simulink model "FP_250521"  (R2024a)
settings: Solver=VariableStepAuto  StartTime=0.0  StopTime=10.0  RelTol=1e-3
values from neighbouring files (symbols this model uses):
  global_path_xy_dense = [-80.8928520527 -80.3602143869 -79.8516651737 -79.3645247642 -78.8961135098 -78.4437517617 -78.004759871 -77.5764581893 -77.1561670675 -76.7412068571 -76.3288979094 -75.9165605754 ... (728 elements, 364x2)]    [global_path_xy_dense_y-34.mat]
undefined symbols (not defined in the file or in its folder): Do_waypoints, do_waypoints_tail_shifted, pathXY, route1_waypoint, route1_waypoint_raw, route2_waypoint, route2_waypoint_raw, route3_waypoint, route3_waypoint_raw
libraries: CarMaker4SL x192, slpidlib x4
(part 2 of 4)

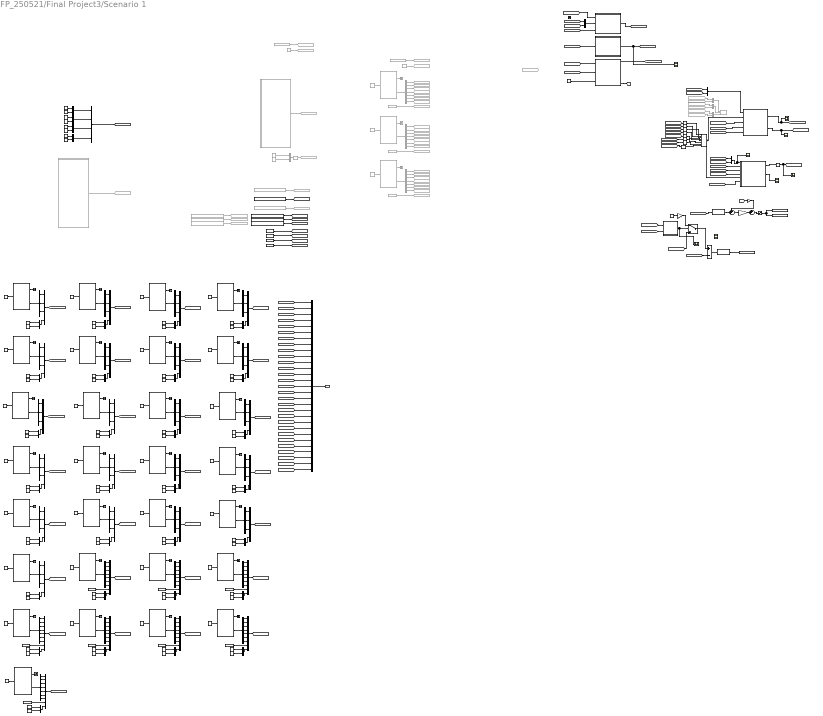
== system FP_250521/Final Project3/Scenario 1 ==
  note: 주차장 들어가기 전, 참이면 1 ==정지
  note: 적분기 출력 제한 -1~1
  note: 주차 경로 개인
  note: 주행 개인
  note: Traffic Size
      | Length: 4.47
      | Width: 1.97
      | Height: 1.12
  note: Traffic Size
      | Length: 4.47
      | Width: 1.97
      | Height: 1.12
  note: Traffic Size
      | Length: 4.47
      | Width: 1.97
      | Height: 1.12
  note: Traffic Size
      | Length: 4.47
      | Width: 1.97
      | Height: 1.12
  note: Traffic Size
      | Length: 4.47
      | Width: 1.97
      | Height: 1.12
  note: Traffic Size
      | Length: 4.47
      | Width: 1.97
      | Height: 1.12
  note: Traffic Size
      | Length: 4.47
      | Width: 1.97
      | Height: 1.12
  note: Traffic Size
      | Length: 4.47
      | Width: 1.97
      | Height: 1.12
  note: Traffic Size
      | Length: 4.47
      | Width: 1.97
      | Height: 1.12
  note: Traffic Size
      | Length: 4.47
      | Width: 1.97
      | Height: 1.12
  note: Traffic Size
      | Length: 4.47
      | Width: 1.97
      | Height: 1.12
  note: Traffic Size
      | Length: 4.47
      | Width: 1.97
      | Height: 1.12
  note: Traffic Size
      | Length: 4.47
      | Width: 1.97
      | Height: 1.12
  note: Traffic Size
      | Length: 4.47
      | Width: 1.97
      | Height: 1.12
  note: Traffic Size
      | Length: 4.47
      | Width: 1.97
      | Height: 1.12
  note: Traffic Size
      | Length: 4.47
      | Width: 1.97
      | Height: 1.12
  note: Traffic Size
      | Length: 4.47
      | Width: 1.97
      | Height: 1.12
  note: Traffic Size
      | Length: 4.47
      | Width: 1.97
      | Height: 1.12
  note: Traffic Size
      | Length: 4.47
      | Width: 1.97
      | Height: 1.12
  note: Traffic Size
      | Length: 4.47
      | Width: 1.97
      | Height: 1.12
  note: Traffic Size
      | Length: 4.47
      | Width: 1.97
      | Height: 1.12
  note: Traffic Size
      | Length: 4.47
      | Width: 1.97
      | Height: 1.12
  note: Traffic Size
      | Length: 4.47
      | Width: 1.97
      | Height: 1.12
  note: Traffic Size
      | Length: 4.47
      | Width: 1.97
      | Height: 1.12
  note: Traffic Size
      | Length: 4.47
      | Width: 1.97
      | Height: 1.12
  note: Traffic Size
      | Length: 4.47
      | Width: 1.97
      | Height: 1.12
  note: Traffic Size
      | Length: 4.47
      | Width: 1.97
      | Height: 1.12
  note: Traffic Size
      | Length: 4.47
      | Width: 1.97
      | Height: 1.12
  note: Traffic Size
      | Length: 4.47
      | Width: 1.97
      | Height: 1.12
  note: Do Not Modify !!
  note: *** Final Project ***
      |
      | Scenario:
      | Input:
      | Output:
      | 제어기 10ms / 다익스트라 1s
  note: Traffic Size
      | Length: 4.47
      | Width: 1.97
      | Height: 1.12
  note: Traffic Size
      | Length: 4.47
      | Width: 1.97
      | Height: 1.12
  note: Modify !!
  note: Traffic Size
      | Length: 4.47
      | Width: 1.97
      | Height: 1.12
  note: Do Not Modify !!
  note: Average Filter
  Add : Sum  Inputs=+-
  Bus Selector : BusSelector  Commented=on  OutputSignals=t_0 x,t_0 y,v_0 x,v_0 y,a_0 x,a_0 y,r_zyx z
  Bus Selector1 : BusSelector  Commented=on  OutputSignals=t_0 x,t_0 y,v_0 x,v_0 y,a_0 x,a_0 y,r_zyx z
  Bus Selector{3..19,22,28..30} (21 alike) : BusSelector  OutputSignals=t_0 x,t_0 y,r_zyx z
  Bus Selector2 : BusSelector  Commented=on  OutputSignals=t_0 x,t_0 y,v_0 x,v_0 y,a_0 x,a_0 y,r_zyx z
  Bus Selector{20..21,23..27,31} (8 alike) : BusSelector  OutputSignals=t_0 x,t_0 y,v_0 x,v_0 y,a_0 x,a_0 y,r_zyx z
  Constant : Constant  Commented=on  Value=80
  Constant1 : Constant  Commented=on  Value=0
  Constant10 : Constant  Commented=on  Value=2.48
  Constant100 : Constant  Value=47.5
  Constant101 : Constant  Value=-45
  Constant102 : Constant  Value=5.5
  Constant103 : Constant  Value=-45
  Constant104 : Constant  Value=47.5
  Constant105 : Constant  Value=-4
  Constant106 : Constant  Commented=on  Value=pathXY
  Constant107 : Constant  Commented=on  Value=route1_waypoint
  Constant108 : Constant  Commented=on  Value=route2_waypoint
  Constant109 : Constant  Commented=on  Value=route3_waypoint
  Constant11 : Constant
  Constant110 : Constant  Value=global_path_xy_dense
  Constant111 : Constant  Commented=on  Value=Do_waypoints
  Constant112 : Constant
  Constant12 : Constant  Value=5
  Constant{13,16,19,21..22,26,29,32,35,39,42,46,48,52,55..56,59,61,65,69,72,74,79,82,85,87..88,92,96} (29 alike) : Constant  Value=4.47
  Constant{14,17,23..24,27,30,33,36..37,40,43,49..50,53,57,62..63,66..67,70,75..76,80,83,89..90,93..94,97} (29 alike) : Constant  Value=1.97
  Constant15 : Constant  Value=7
  Constant18 : Constant  Value=8
  Constant2 : Constant  Commented=on
  Constant20 : Constant  Value=4
  Constant25 : Constant  Value=10
  Constant28 : Constant  Value=11
  Constant3 : Constant  Commented=on  Value=2
  Constant31 : Constant  Value=12
  Constant34 : Constant  Value=9
  Constant38 : Constant  Value=14
  Constant4 : Constant  Commented=on  Value=80
  Constant41 : Constant  Value=15
  Constant44 : Constant  Value=2
  Constant45 : Constant  Value=16
  Constant47 : Constant  Value=13
  Constant5 : Constant  Commented=on  Value=11.5
  Constant51 : Constant  Value=18
  Constant54 : Constant  Value=19
  Constant58 : Constant  Value=6
  Constant6 : Constant  Value=route1_waypoint_raw
  Constant60 : Constant  Value=17
  Constant64 : Constant  Value=21
  Constant68 : Constant  Value=22
  Constant7 : Constant
  Constant71 : Constant  Value=23
  Constant73 : Constant  Value=20
  Constant77 : Constant  Value=3
  Constant78 : Constant  Value=25
  Constant8 : Constant  Value=route2_waypoint_raw
  Constant81 : Constant  Value=26
  Constant84 : Constant  Value=27
  Constant86 : Constant  Value=24
  Constant9 : Constant  Value=route3_waypoint_raw
  Constant91 : Constant  Value=0
  Constant95 : Constant  Value=28
  Constant98 : Constant  Value=5.5
  Constant99 : Constant  Value=-4
  From2 : From  Commented=on  GotoTag=Global_Waypoints2
  From28 : From  Commented=on  GotoTag=Traffic00_Global_X
  From29 : From  Commented=on  GotoTag=Traffic00_Global_Y
  From30 : From  Commented=on  GotoTag=Traffic01_Global_X
  From31 : From  Commented=on  GotoTag=Traffic01_Global_Y
  From32 : From  Commented=on  GotoTag=Traffic02_Global_X
  From33 : From  Commented=on  GotoTag=Traffic02_Global_Y
  Gain : Gain  Gain=pi/180
  Gain1 : Gain  Gain=3
  Gain2 : Gain  Gain=0
  Goto1 : Goto  Commented=on  GotoTag=CrossTrackError
  Goto10 : Goto  Commented=on  GotoTag=Traffic00_Yaw
  Goto11 : Goto  Commented=on  GotoTag=Traffic01_Yaw
  Goto12 : Goto  Commented=on  GotoTag=Traffic01_YawRate
  Goto13 : Goto  Commented=on  GotoTag=Traffic01_Global_X
  Goto14 : Goto  Commented=on  GotoTag=Traffic01_Global_Y
  Goto15 : Goto  Commented=on  GotoTag=Traffic01_Vx
  Goto16 : Goto  Commented=on  GotoTag=Traffic01_Vy
  Goto17 : Goto  Commented=on  GotoTag=Traffic01_Ax
  Goto18 : Goto  Commented=on  GotoTag=Traffic01_Ay
  Goto19 : Goto  Commented=on  GotoTag=Traffic02_Yaw
  Goto2 : Goto  Commented=on  GotoTag=Traffic00_YawRate
  Goto20 : Goto  Commented=on  GotoTag=Traffic02_YawRate
  Goto21 : Goto  Commented=on  GotoTag=Traffic02_Global_X
  Goto22 : Goto  Commented=on  GotoTag=Traffic02_Global_Y
  Goto23 : Goto  Commented=on  GotoTag=Traffic02_Vx
  Goto24 : Goto  Commented=on  GotoTag=Traffic02_Vy
  Goto25 : Goto  Commented=on  GotoTag=Traffic02_Ax
  Goto26 : Goto  Commented=on  GotoTag=Traffic02_Ay
  Goto27 : Goto  Commented=on  GotoTag=CrossTrackError
  Goto28 : Goto  Commented=on  GotoTag=Traffic_size
  Goto29 : Goto  Commented=on  GotoTag=Target_Speed
  Goto3 : Goto  Commented=on  GotoTag=Traffic00_Global_X
  Goto30 : Goto  Commented=on  GotoTag=Traffic_Info
  Goto4 : Goto  Commented=on  GotoTag=Target_Speed
  Goto5 : Goto  Commented=on  GotoTag=Traffic00_Global_Y
  Goto6 : Goto  Commented=on  GotoTag=Traffic00_Vx
  Goto7 : Goto  Commented=on  GotoTag=Traffic00_Vy
  Goto73 : Goto  Commented=on  GotoTag=Global_Waypoints4
  Goto75 : Goto  Commented=on  GotoTag=Obstacle_Info
  Goto76 : Goto  Commented=on  GotoTag=Global_Waypoints1
  Goto77 : Goto  Commented=on  GotoTag=Global_Waypoints2
  Goto78 : Goto  Commented=on  GotoTag=Global_Waypoints3
  Goto8 : Goto  Commented=on  GotoTag=Traffic00_Ax
  Goto80 : Goto  Commented=on  GotoTag=Global_Waypoints4
  Goto9 : Goto  Commented=on  GotoTag=Traffic00_Ay
  Ground : Ground
  MATLAB Function : MATLAB Function  TreatAsAtomicUnit=on
  MATLAB Function11 : MATLAB Function  TreatAsAtomicUnit=on
  MATLAB Function3 : MATLAB Function  TreatAsAtomicUnit=on
  MATLAB Function4 : MATLAB Function  TreatAsAtomicUnit=on
  "MATLAB Function4 " : MATLAB Function  TreatAsAtomicUnit=on
  MATLAB Function9 : MATLAB Function  TreatAsAtomicUnit=on
  Matrix Concatenate : Concatenate  NumInputs=8  Mode=Multidimensional array
  Matrix Concatenate1 : Concatenate  Commented=on  NumInputs=3  Mode=Multidimensional array
  Mux{,2,4,6,8,11,13,15,17,19,21,23,25,27,29,31,33,35,37,39,41,43,45,47,49,51,53,55..56,58,61,63,65,67..69} (36 alike) : Mux  Inputs=2
  Mux{1,5,9..10,12,14,16,18,20,22,24,26,28,30,32,34,36,38,46,57,60,66} (22 alike) : Mux
  Mux3 : Mux  Commented=on  Inputs=2
  Mux{40,42,44,48,50,52,54,64} (8 alike) : Mux  Inputs=9
  Mux59 : Mux  Inputs=29
  PID Controller : slpidlib/PID Controller  Controller=PID  Form=Ideal  TimeDomain=Discrete-time  UseExternalTs=off  SampleTime=-1  IntegratorMethod=Forward Euler  FilterMethod=Forward Euler  ControllerParametersSource=internal  P=5  I=0.25  UseKiTs=off  D=2.8  UseExternalDerivativeSource=off  N=1000  UseFilter=off  TunerSelectOption=Transfer Function Based (PID Tuner App)  InitialConditionSource=internal  InitialConditionForIntegrator=0  InitialConditionForFilter=0  DifferentiatorICPrevScaledInput=0  ExternalReset=none  TrackingMode=off  Kt=1  LimitOutput=off  SatLimitsSource=internal  UpperSaturationLimit=1  LowerSaturationLimit=-1  LinearizeAsGain=on  AntiWindupMode=back-calculation  Kb=1  LimitIntegrator=on  UpperIntegratorSaturationLimit=1  LowerIntegratorSaturationLimit=-1  POutMin=[]  POutMax=[]  IOutMin=[]  IOutMax=[]  DOutMin=[]  DOutMax=[]  NOutMin=[]  NOutMax=[]  SumOutMin=[]  SumOutMax=[]  SaturationOutMin=[]  SaturationOutMax=[]  PParamMin=[]  PParamMax=[]  IParamMin=[]  IParamMax=[]  DParamMin=[]  DParamMax=[]  NParamMin=[]  NParamMax=[]  KbParamMin=[]  KbParamMax=[]  KtParamMin=[]  KtParamMax=[]  KbOutMin=[]  KbOutMax=[]  KtOutMin=[]  KtOutMax=[]  IntegratorOutMin=[]  IntegratorOutMax=[]  FilterOutMin=[]  FilterOutMax=[]  SumI1OutMin=[]  SumI1OutMax=[]  SumI2OutMin=[]  SumI2OutMax=[]  SumI3OutMin=[]  SumI3OutMax=[]  SumI4OutMin=[]  SumI4OutMax=[]  SumDOutMin=[]  SumDOutMax=[]  DifferentiatorOutMin=[]  DifferentiatorOutMax=[]  FilterDiffOutCoefMin=[]  FilterDiffOutCoefMax=[]  ReciprocalOutMin=[]  ReciprocalOutMax=[]  SumDenOutMin=[]  SumDenOutMax=[]  SumNumOutMin=[]  SumNumOutMax=[]  DivideOutMin=[]  DivideOutMax=[]  UdiffTsProdOutMin=[]  UdiffTsProdOutMax=[]  NTsProdOutMin=[]  NTsProdOutMax=[]  UintegralTsProdOutMin=[]  UintegralTsProdOutMax=[]  UngainTsProdOutMin=[]  UngainTsProdOutMax=[]  ClampingZeroOutDataTypeStr=Inherit: Inherit via back propagation  ClampingZeroOutMin=[]  ClampingZeroOutMax=[]  FilterDenConstantOutDataTypeStr=Inherit: Inherit via back propagation  FilterDenConstantOutMin=[]  FilterDenConstantOutMax=[]  PCopyOutDataTypeStr=Inherit: Inherit via back propagation  PCopyOutMin=[]  PCopyOutMax=[]  NCopyOutDataTypeStr=Inherit: Inherit via back propagation  NCopyOutMin=[]  NCopyOutMax=[]  IntegratorContinuousStateAttributes=''  IntegratorStateMustResolveToSignalObject=off  IntegratorRTWStateStorageClass=Auto  FilterContinuousStateAttributes=''  FilterStateMustResolveToSignalObject=off  FilterRTWStateStorageClass=Auto  ParallelPVariant=Passthrough  IdealPVariant=InternalParameters  IVariant=InternalParameters  DVariant=InternalParameters  IntegratorVariant=Discrete  SatVariant=Disabled  AWVariant=Passthrough  PCopyVariant=Disabled  TRVariant=Disabled  FdbkBlocksVariant=Forward  IdealPFdbkVariant=Disabled  SatFdbkVariant=Disabled  DerivativeFilterVariant=Differentiator  NVariant=Passthrough  NCopyVariant=Disabled_SignalSpec  FilterICVariant=InternalICsDifferentiator  IntegratorICVariant=InternalICs  ExternalResetVariant=Disabled  TRSumVariant=Passthrough  SumFdbkVariant=Disabled  SumVariant=Sum_PID  TsampFilterVariant=InternalTs  TsampNgainVariant=Passthrough  TsampIntegralVariant=Disabled_SignalSpec  ExternalSaturationOutDataTypeStr=Inherit: Same as second input  DerivativeSourceVariant=ErrorSignal
  PID Controller1 : slpidlib/PID Controller  Controller=PID  Form=Ideal  TimeDomain=Discrete-time  UseExternalTs=off  SampleTime=-1  IntegratorMethod=Forward Euler  FilterMethod=Forward Euler  ControllerParametersSource=internal  P=3  I=0  UseKiTs=off  D=0.1  UseExternalDerivativeSource=off  N=1000  UseFilter=off  TunerSelectOption=Transfer Function Based (PID Tuner App)  InitialConditionSource=internal  InitialConditionForIntegrator=0  InitialConditionForFilter=0  DifferentiatorICPrevScaledInput=0  ExternalReset=none  TrackingMode=off  Kt=1  LimitOutput=off  SatLimitsSource=internal  UpperSaturationLimit=1  LowerSaturationLimit=-1  LinearizeAsGain=on  AntiWindupMode=back-calculation  Kb=1  LimitIntegrator=off  UpperIntegratorSaturationLimit=0.7  LowerIntegratorSaturationLimit=-0.7  POutMin=[]  POutMax=[]  IOutMin=[]  IOutMax=[]  DOutMin=[]  DOutMax=[]  NOutMin=[]  NOutMax=[]  SumOutMin=[]  SumOutMax=[]  SaturationOutMin=[]  SaturationOutMax=[]  PParamMin=[]  PParamMax=[]  IParamMin=[]  IParamMax=[]  DParamMin=[]  DParamMax=[]  NParamMin=[]  NParamMax=[]  KbParamMin=[]  KbParamMax=[]  KtParamMin=[]  KtParamMax=[]  KbOutMin=[]  KbOutMax=[]  KtOutMin=[]  KtOutMax=[]  IntegratorOutMin=[]  IntegratorOutMax=[]  FilterOutMin=[]  FilterOutMax=[]  SumI1OutMin=[]  SumI1OutMax=[]  SumI2OutMin=[]  SumI2OutMax=[]  SumI3OutMin=[]  SumI3OutMax=[]  SumI4OutMin=[]  SumI4OutMax=[]  SumDOutMin=[]  SumDOutMax=[]  DifferentiatorOutMin=[]  DifferentiatorOutMax=[]  FilterDiffOutCoefMin=[]  FilterDiffOutCoefMax=[]  ReciprocalOutMin=[]  ReciprocalOutMax=[]  SumDenOutMin=[]  SumDenOutMax=[]  SumNumOutMin=[]  SumNumOutMax=[]  DivideOutMin=[]  DivideOutMax=[]  UdiffTsProdOutMin=[]  UdiffTsProdOutMax=[]  NTsProdOutMin=[]  NTsProdOutMax=[]  UintegralTsProdOutMin=[]  UintegralTsProdOutMax=[]  UngainTsProdOutMin=[]  UngainTsProdOutMax=[]  ClampingZeroOutDataTypeStr=Inherit: Inherit via back propagation  ClampingZeroOutMin=[]  ClampingZeroOutMax=[]  FilterDenConstantOutDataTypeStr=Inherit: Inherit via back propagation  FilterDenConstantOutMin=[]  FilterDenConstantOutMax=[]  PCopyOutDataTypeStr=Inherit: Inherit via back propagation  PCopyOutMin=[]  PCopyOutMax=[]  NCopyOutDataTypeStr=Inherit: Inherit via back propagation  NCopyOutMin=[]  NCopyOutMax=[]  IntegratorContinuousStateAttributes=''  IntegratorStateMustResolveToSignalObject=off  IntegratorRTWStateStorageClass=Auto  FilterContinuousStateAttributes=''  FilterStateMustResolveToSignalObject=off  FilterRTWStateStorageClass=Auto  ParallelPVariant=Passthrough  IdealPVariant=InternalParameters  IVariant=InternalParameters  DVariant=InternalParameters  IntegratorVariant=Discrete  SatVariant=Disabled  AWVariant=Passthrough  PCopyVariant=Disabled  TRVariant=Disabled  FdbkBlocksVariant=Forward  IdealPFdbkVariant=Disabled  SatFdbkVariant=Disabled  DerivativeFilterVariant=Differentiator  NVariant=Passthrough  NCopyVariant=Disabled_SignalSpec  FilterICVariant=InternalICsDifferentiator  IntegratorICVariant=InternalICs  ExternalResetVariant=Disabled  TRSumVariant=Passthrough  SumFdbkVariant=Disabled  SumVariant=Sum_PID  TsampFilterVariant=InternalTs  TsampNgainVariant=Passthrough  TsampIntegralVariant=Disabled_SignalSpec  ExternalSaturationOutDataTypeStr=Inherit: Same as second input  DerivativeSourceVariant=ErrorSignal
  Rate Limiter : RateLimiter  RisingSlewLimit=1.1  FallingSlewLimit=-3.0  SampleTimeMode=inherited  InitialCondition=13.0
  Read CM Dict : CarMaker4SL/Read CM Dict  Commented=on  xname=Car.Road.Path.DevDist  xsync=off  xstime=Inherited
  Read CM Dict1 : CarMaker4SL/Read CM Dict  Commented=on  xname=Traffic.T22.rzv  xsync=off  xstime=Inherited
  Read CM Dict2 : CarMaker4SL/Read CM Dict  Commented=on  xname=Traffic.T23.rzv  xsync=off  xstime=Inherited
  Read CM Dict22 : CarMaker4SL/Read CM Dict  xname=Traffic.T21.rzv  xsync=off  xstime=Inherited
  Read CM Dict23 : CarMaker4SL/Read CM Dict  xname=Traffic.T22.rzv  xsync=off  xstime=Inherited
  Read CM Dict24 : CarMaker4SL/Read CM Dict  xname=Traffic.T23.rzv  xsync=off  xstime=Inherited
  Read CM Dict25 : CarMaker4SL/Read CM Dict  xname=Traffic.T24.rzv  xsync=off  xstime=Inherited
  Read CM Dict26 : CarMaker4SL/Read CM Dict  xname=Traffic.T25.rzv  xsync=off  xstime=Inherited
  Read CM Dict27 : CarMaker4SL/Read CM Dict  xname=Traffic.T26.rzv  xsync=off  xstime=Inherited
  Read CM Dict28 : CarMaker4SL/Read CM Dict  xname=Traffic.T27.rzv  xsync=off  xstime=Inherited
  Read CM Dict29 : CarMaker4SL/Read CM Dict  xname=Traffic.T28.rzv  xsync=off  xstime=Inherited
  Read CM Dict3 : CarMaker4SL/Read CM Dict  Commented=on  xname=Traffic.T24.rzv  xsync=off  xstime=Inherited
  Read CM Dict4 : CarMaker4SL/Read CM Dict  Commented=on  xname=Car.Road.Path.DevDist  xsync=off  xstime=Inherited
  Read CM Dict5 : CarMaker4SL/Read CM Dict  xname=Car.Fr1.tx  xsync=off  xstime=Inherited
  Read CM Dict6 : CarMaker4SL/Read CM Dict  xname=Car.Fr1.ty  xsync=off  xstime=Inherited
  Read CM Dict7 : CarMaker4SL/Read CM Dict  xname=Car.v  xsync=off  xstime=Inherited
  Read CM Dict8 : CarMaker4SL/Read CM Dict  xname=Car.Fr1.rz  xsync=off  xstime=Inherited
  Reshape1 : Reshape  Commented=on  OutputDimensionality=Row vector (2-D)  OutputDimensions=[2,2]
  Saturation1 : Saturate  UpperLimit=2  LowerLimit=-2
  Scope{,1..6,8} (8 alike) : Scope
  Subsystem : Subsystem  Commented=on
  Subsystem1 : Subsystem  Commented=on
  Sum : Sum  Inputs=++|
  Sum1 : Sum  Inputs=++|
  Switch : Switch  Threshold=1  SaturateOnIntegerOverflow=off  InputSameDT=off
  Terminator : Terminator  Commented=on
  Terminator1 : Terminator  Commented=on
  Terminator{3..31} (29 alike) : Terminator
  Terminator2 : Terminator  Commented=on
  Traffic Object : CarMaker4SL/Traffic Object  Commented=on  xname=T00  ximode=Traffic Id  xstime=Inherited
      settings: SourceProductName=CarMaker4SL
  Traffic Object1 : CarMaker4SL/Traffic Object  Commented=on  xname=T01  ximode=Traffic Id  xstime=Inherited
      settings: SourceProductName=CarMaker4SL
  Traffic Object10 : CarMaker4SL/Traffic Object  xname=T11  ximode=Traffic Id  xstime=Inherited
      settings: SourceProductName=CarMaker4SL
  Traffic Object11 : CarMaker4SL/Traffic Object  xname=T12  ximode=Traffic Id  xstime=Inherited
      settings: SourceProductName=CarMaker4SL
  Traffic Object12 : CarMaker4SL/Traffic Object  xname=T13  ximode=Traffic Id  xstime=Inherited
      settings: SourceProductName=CarMaker4SL
  Traffic Object13 : CarMaker4SL/Traffic Object  xname=T14  ximode=Traffic Id  xstime=Inherited
      settings: SourceProductName=CarMaker4SL
  Traffic Object14 : CarMaker4SL/Traffic Object  xname=T15  ximode=Traffic Id  xstime=Inherited
      settings: SourceProductName=CarMaker4SL
  Traffic Object15 : CarMaker4SL/Traffic Object  xname=T16  ximode=Traffic Id  xstime=Inherited
      settings: SourceProductName=CarMaker4SL
  Traffic Object16 : CarMaker4SL/Traffic Object  xname=T17  ximode=Traffic Id  xstime=Inherited
      settings: SourceProductName=CarMaker4SL
  Traffic Object17 : CarMaker4SL/Traffic Object  xname=T18  ximode=Traffic Id  xstime=Inherited
      settings: SourceProductName=CarMaker4SL
  Traffic Object18 : CarMaker4SL/Traffic Object  xname=T19  ximode=Traffic Id  xstime=Inherited
      settings: SourceProductName=CarMaker4SL
  Traffic Object19 : CarMaker4SL/Traffic Object  xname=T06  ximode=Traffic Id  xstime=Inherited
      settings: SourceProductName=CarMaker4SL
  Traffic Object2 : CarMaker4SL/Traffic Object  Commented=on  xname=T02  ximode=Traffic Id  xstime=Inherited
      settings: SourceProductName=CarMaker4SL
  Traffic Object20 : CarMaker4SL/Traffic Object  xname=T20  ximode=Traffic Id  xstime=Inherited
      settings: SourceProductName=CarMaker4SL
  Traffic Object21 : CarMaker4SL/Traffic Object  xname=T21  ximode=Traffic Id  xstime=Inherited
      settings: SourceProductName=CarMaker4SL
  Traffic Object22 : CarMaker4SL/Traffic Object  xname=T22  ximode=Traffic Id  xstime=Inherited
      settings: SourceProductName=CarMaker4SL
  Traffic Object23 : CarMaker4SL/Traffic Object  xname=T23  ximode=Traffic Id  xstime=Inherited
      settings: SourceProductName=CarMaker4SL
  Traffic Object24 : CarMaker4SL/Traffic Object  xname=T24  ximode=Traffic Id  xstime=Inherited
      settings: SourceProductName=CarMaker4SL
  Traffic Object25 : CarMaker4SL/Traffic Object  xname=T25  ximode=Traffic Id  xstime=Inherited
      settings: SourceProductName=CarMaker4SL
  Traffic Object26 : CarMaker4SL/Traffic Object  xname=T26  ximode=Traffic Id  xstime=Inherited
      settings: SourceProductName=CarMaker4SL
  Traffic Object27 : CarMaker4SL/Traffic Object  xname=T27  ximode=Traffic Id  xstime=Inherited
      settings: SourceProductName=CarMaker4SL
  Traffic Object28 : CarMaker4SL/Traffic Object  xname=T28  ximode=Traffic Id  xstime=Inherited
      settings: SourceProductName=CarMaker4SL
  Traffic Object29 : CarMaker4SL/Traffic Object  xname=T08  ximode=Traffic Id  xstime=Inherited
      settings: SourceProductName=CarMaker4SL
  Traffic Object3 : CarMaker4SL/Traffic Object  xname=T00  ximode=Traffic Id  xstime=Inherited
      settings: SourceProductName=CarMaker4SL
  Traffic Object30 : CarMaker4SL/Traffic Object  xname=T09  ximode=Traffic Id  xstime=Inherited
      settings: SourceProductName=CarMaker4SL
  Traffic Object31 : CarMaker4SL/Traffic Object  xname=T10  ximode=Traffic Id  xstime=Inherited
      settings: SourceProductName=CarMaker4SL
  Traffic Object4 : CarMaker4SL/Traffic Object  xname=T01  ximode=Traffic Id  xstime=Inherited
      settings: SourceProductName=CarMaker4SL
  Traffic Object5 : CarMaker4SL/Traffic Object  xname=T02  ximode=Traffic Id  xstime=Inherited
      settings: SourceProductName=CarMaker4SL
  Traffic Object6 : CarMaker4SL/Traffic Object  xname=T03  ximode=Traffic Id  xstime=Inherited
      settings: SourceProductName=CarMaker4SL
  Traffic Object7 : CarMaker4SL/Traffic Object  xname=T04  ximode=Traffic Id  xstime=Inherited
      settings: SourceProductName=CarMaker4SL
  Traffic Object8 : CarMaker4SL/Traffic Object  xname=T05  ximode=Traffic Id  xstime=Inherited
      settings: SourceProductName=CarMaker4SL
  Traffic Object9 : CarMaker4SL/Traffic Object  xname=T07  ximode=Traffic Id  xstime=Inherited
      settings: SourceProductName=CarMaker4SL
  Transpose{,1..7} (8 alike) : Math  Operator=transpose
  Vector Concatenate3 : Concatenate  Commented=on  Mode=Multidimensional array  ConcatenateDimension=2
  Vector Concatenate4 : Concatenate  Commented=on  Mode=Multidimensional array  ConcatenateDimension=2
  Vector Concatenate5 : Concatenate  Commented=on  Mode=Multidimensional array  ConcatenateDimension=2
  Write CM Dict3 : CarMaker4SL/Write CM Dict  xname=Car.CFL.rz_ext  xsync=off
  Write CM Dict4 : CarMaker4SL/Write CM Dict  xname=Car.CFR.rz_ext  xsync=off
  Write CM Dict5 : CarMaker4SL/Write CM Dict  xname=AccelCtrl.DesiredAx  xsync=off
  Traffic_Info : Outport
  wires:
  Constant111/1 -> Goto80/1
  Sum1/1 -> Gain/1
  PID Controller/1 -> Sum1/2
  [delta] -> Gain1/1
  Sum/1 -> Saturation1/1
  Gain/1 -> Sum/2
  MATLAB Function3/6(kappa) -> [delta]
  Constant110/1 -> [Global_Waypoints4]
  Constant107/1 -> Goto76/1
  Constant108/1 -> Goto77/1
  Constant109/1 -> Goto78/1
  [LateralError] -> PID Controller/1
  Constant106/1 -> Goto73/1
  Transpose5/1 -> Matrix Concatenate/6
  Transpose7/1 -> Matrix Concatenate/8
  Transpose6/1 -> Matrix Concatenate/7
  Transpose4/1 -> Matrix Concatenate/5
  Transpose3/1 -> Matrix Concatenate/4
  Transpose2/1 -> Matrix Concatenate/3
  Transpose1/1 -> Matrix Concatenate/2
  Transpose/1 -> Matrix Concatenate/1
  [Traffic_Info_26] -> Mux59/27
  Constant35/1 -> Mux23/1
  Constant79/1 -> Mux49/1
  Traffic Object31/1 -> Terminator31/1
  [Traffic_Info_22] -> Mux59/23
  Bus Selector14/2 -> Mux30/2  "<t_0 y>"
  Mux1/1 -> [Traffic_Info_01]
  Bus Selector17/1 -> Mux34/1  "<t_0 x>"
  Mux18/1 -> [Traffic_Info_11]
  Bus Selector26/3 -> Mux54/3  "<v_0 x>"
  Constant97/1 -> Mux65/2
  Bus Selector24/7 -> Mux48/7  "<r_zyx z>"
  Bus Selector16/3 -> Mux32/3  "<r_zyx z>"
  Constant33/1 -> Mux4/2
  Constant68/1 -> Traffic Object22/1
  Bus Selector5/3 -> Mux9/3  "<r_zyx z>"
  Bus Selector19/3 -> Mux36/3  "<r_zyx z>"
  Bus Selector14/1 -> Mux30/1  "<t_0 x>"
  Mux49/1 -> Mux48/9
  Read CM Dict27/1 -> Mux50/8
  Bus Selector25/6 -> Mux50/6  "<a_0 y>"
  Mux25/1 -> Mux24/4
  Constant59/1 -> Mux37/1
  Constant62/1 -> Mux37/2
  [Traffic_Info_14] -> Mux59/15
  Bus Selector23/1 -> Mux44/1  "<t_0 x>"
  Constant39/1 -> Mux25/1
  Constant55/1 -> Mux8/1
  Bus Selector25/4 -> Mux50/4  "<v_0 y>"
  Bus Selector22/1 -> Mux46/1  "<t_0 x>"
  Bus Selector21/4 -> Mux42/4  "<v_0 y>"
  Mux32/1 -> [Traffic_Info_18]
  Constant84/1 -> Traffic Object27/1
  Mux12/1 -> [Traffic_Info_08]
  Constant73/1 -> Traffic Object20/1
  Bus Selector23/2 -> Mux44/2  "<t_0 y>"
  Bus Selector26/5 -> Mux54/5  "<a_0 x>"
  Mux37/1 -> Mux36/4
  Traffic Object18/1 -> Terminator18/1
  Bus Selector23/7 -> Mux44/7  "<r_zyx z>"
  Bus Selector31/4 -> Mux64/4  "<v_0 y>"
  Mux45/1 -> Mux44/9
  Traffic Object13/1 -> Terminator13/1
  Traffic Object26/2 -> Bus Selector25/1
  Traffic Object24/2 -> Bus Selector26/1
  Constant58/1 -> Traffic Object19/1
  Traffic Object19/1 -> Terminator19/1
  Traffic Object3/2 -> Bus Selector29/1
  Constant27/1 -> Mux17/2
  Bus Selector15/2 -> Mux28/2  "<t_0 y>"
  Bus Selector19/2 -> Mux36/2  "<t_0 y>"
  [Traffic_Info_10] -> Mux59/11
  Bus Selector4/2 -> Mux5/2  "<t_0 y>"
  Constant76/1 -> Mux47/2
  Mux22/1 -> [Traffic_Info_09]
  Mux43/1 -> Mux42/9
  Mux26/1 -> [Traffic_Info_15]
  Constant30/1 -> Mux19/2
  Traffic Object13/2 -> Bus Selector12/1
  Bus Selector24/3 -> Mux48/3  "<v_0 x>"
  Bus Selector29/3 -> Mux60/3  "<r_zyx z>"
  Mux60/1 -> [Traffic_Info_00]
  Constant92/1 -> Mux61/1
  Traffic Object25/2 -> Bus Selector24/1
  Traffic Object22/2 -> Bus Selector21/1
  Read CM Dict22/1 -> Mux40/8
  Mux10/1 -> [Traffic_Info_07]
  Constant70/1 -> Mux43/2
  Traffic Object23/1 -> Terminator23/1
  Bus Selector28/2 -> Mux16/2  "<t_0 y>"
  Constant75/1 -> Mux45/2
  Traffic Object14/2 -> Bus Selector13/1
  Bus Selector21/5 -> Mux42/5  "<a_0 x>"
  Constant83/1 -> Mux51/2
  Mux40/1 -> [Traffic_Info_21]
  Traffic Object20/2 -> Bus Selector22/1
  Mux35/1 -> Mux34/4
  Constant93/1 -> Mux56/2
  Mux11/1 -> Mux10/4
  Bus Selector21/6 -> Mux42/6  "<a_0 y>"
  [Traffic_Info_16] -> Mux59/17
  Bus Selector20/6 -> Mux40/6  "<a_0 y>"
  Constant94/1 -> Mux61/2
  Mux55/1 -> Mux54/9
  Bus Selector23/4 -> Mux44/4  "<v_0 y>"
  Constant69/1 -> Mux43/1
  Mux36/1 -> [Traffic_Info_06]
  Bus Selector10/3 -> Mux22/3  "<r_zyx z>"
  Mux57/1 -> [Traffic_Info_05]
  Mux59/1 -> Traffic_Info/1
  [Traffic_Info_08] -> Mux59/9
  Constant64/1 -> Traffic Object21/1
  Traffic Object6/1 -> Terminator6/1
  Constant50/1 -> Mux31/2
  Mux51/1 -> Mux50/9
  Bus Selector21/7 -> Mux42/7  "<r_zyx z>"
  Traffic Object27/1 -> Terminator27/1
  Bus Selector20/1 -> Mux40/1  "<t_0 x>"
  Constant25/1 -> Traffic Object31/1
  Constant72/1 -> Mux45/1
  Bus Selector29/2 -> Mux60/2  "<t_0 y>"
  Traffic Object22/1 -> Terminator22/1
  Constant71/1 -> Traffic Object23/1
  Bus Selector20/5 -> Mux40/5  "<a_0 x>"
  Constant43/1 -> Mux27/2
  Constant29/1 -> Mux19/1
  Traffic Object21/1 -> Terminator21/1
  Read CM Dict23/1 -> Mux42/8
  Bus Selector24/1 -> Mux48/1  "<t_0 x>"
  Bus Selector20/7 -> Mux40/7  "<r_zyx z>"
  Bus Selector7/1 -> Mux10/1  "<t_0 x>"
  Bus Selector26/6 -> Mux54/6  "<a_0 y>"
  [Traffic_Info_11] -> Mux59/12
  [Traffic_Info_18] -> Mux59/19
  Bus Selector20/4 -> Mux40/4  "<v_0 y>"
  Mux54/1 -> [Traffic_Info_24]
  Bus Selector25/5 -> Mux50/5  "<a_0 x>"
  Bus Selector3/1 -> Mux1/1  "<t_0 x>"
  Bus Selector27/2 -> Mux52/2  "<t_0 y>"
  Bus Selector21/3 -> Mux42/3  "<v_0 x>"
  Traffic Object11/2 -> Bus Selector11/1
  Bus Selector25/2 -> Mux50/2  "<t_0 y>"
  Traffic Object15/1 -> Terminator15/1
  Bus Selector27/5 -> Mux52/5  "<a_0 x>"
  Bus Selector22/3 -> Mux46/3  "<r_zyx z>"
  Traffic Object26/1 -> Terminator26/1
  Read CM Dict24/1 -> Mux44/8
  Bus Selector26/7 -> Mux54/7  "<r_zyx z>"
  [Traffic_Info_23] -> Mux59/24
  Bus Selector23/3 -> Mux44/3  "<v_0 x>"
  Traffic Object24/1 -> Terminator24/1
  Traffic Object12/1 -> Terminator12/1
  Traffic Object4/2 -> Bus Selector3/1
  Read CM Dict28/1 -> Mux52/8
  Mux53/1 -> Mux52/9
  Mux52/1 -> [Traffic_Info_27]
  Bus Selector25/1 -> Mux50/1  "<t_0 x>"
  Bus Selector26/4 -> Mux54/4  "<v_0 y>"
  Constant86/1 -> Traffic Object24/1
  Mux28/1 -> [Traffic_Info_16]
  Constant24/1 -> Mux15/2
  Bus Selector27/4 -> Mux52/4  "<v_0 y>"
  Bus Selector24/6 -> Mux48/6  "<a_0 y>"
  [Traffic_Info_06] -> Mux59/7
  Constant96/1 -> Mux65/1
  [Traffic_Info_19] -> Mux59/20
  Constant78/1 -> Traffic Object25/1
  Bus Selector27/7 -> Mux52/7  "<r_zyx z>"
  Constant67/1 -> Mux41/2
  Read CM Dict25/1 -> Mux54/8
  Constant57/1 -> Mux35/2
  Mux24/1 -> [Traffic_Info_14]
  [Traffic_Info_04] -> Mux59/5
  Bus Selector24/2 -> Mux48/2  "<t_0 y>"
  Bus Selector7/3 -> Mux10/3  "<r_zyx z>"
  Bus Selector25/7 -> Mux50/7  "<r_zyx z>"
  Constant82/1 -> Mux51/1
  Traffic Object25/1 -> Terminator25/1
  Mux41/1 -> Mux40/9
  Bus Selector22/2 -> Mux46/2  "<t_0 y>"
  Constant80/1 -> Mux49/2
  Bus Selector31/7 -> Mux64/7  "<r_zyx z>"
  Constant45/1 -> Traffic Object15/1
  Constant89/1 -> Mux53/2
  Constant90/1 -> Mux55/2
  Bus Selector13/2 -> Mux26/2  "<t_0 y>"
  Bus Selector31/1 -> Mux64/1  "<t_0 x>"
  Constant87/1 -> Mux55/1
  Traffic Object28/1 -> Terminator28/1
  Constant74/1 -> Mux47/1
  Traffic Object4/1 -> Terminator4/1
  Traffic Object12/2 -> Bus Selector14/1
  Mux14/1 -> [Traffic_Info_04]
  [Traffic_Info_12] -> Mux59/13
  Constant11/1 -> Traffic Object4/1
  Bus Selector3/2 -> Mux1/2  "<t_0 y>"
  Constant47/1 -> Traffic Object12/1
  Bus Selector31/2 -> Mux64/2  "<t_0 y>"
  Traffic Object28/2 -> Bus Selector31/1
  Traffic Object5/1 -> Terminator5/1
  Read CM Dict29/1 -> Mux64/8
  [Traffic_Info_24] -> Mux59/25
  Mux8/1 -> Mux5/4
  Bus Selector23/5 -> Mux44/5  "<a_0 x>"
  Constant44/1 -> Traffic Object5/1
  [Traffic_Info_01] -> Mux59/2
  Mux64/1 -> [Traffic_Info_28]
  Traffic Object6/2 -> Bus Selector5/1
  Bus Selector15/1 -> Mux28/1  "<t_0 x>"
  Mux58/1 -> Mux57/4
  [Traffic_Info_25] -> Mux59/26
  Bus Selector5/1 -> Mux9/1  "<t_0 x>"
  Mux56/1 -> Mux9/4
  Constant14/1 -> Mux58/2
  Bus Selector31/3 -> Mux64/3  "<v_0 x>"
  [Traffic_Info_05] -> Mux59/6
  Bus Selector8/3 -> Mux14/3  "<r_zyx z>"
  Constant12/1 -> Traffic Object8/1
  Constant85/1 -> Mux53/1
  Constant53/1 -> Mux33/2
  Mux61/1 -> Mux60/4
  Bus Selector5/2 -> Mux9/2  "<t_0 y>"
  Constant48/1 -> Mux31/1
  Mux9/1 -> [Traffic_Info_03]
  Bus Selector24/5 -> Mux48/5  "<a_0 x>"
  Constant18/1 -> Traffic Object29/1
  Constant60/1 -> Traffic Object16/1
  Bus Selector30/1 -> Mux18/1  "<t_0 x>"
  Mux15/1 -> Mux14/4
  Constant28/1 -> Traffic Object10/1
  Bus Selector6/2 -> Mux57/2  "<t_0 y>"
  Constant13/1 -> Mux58/1
  Constant65/1 -> Mux41/1
  Bus Selector20/3 -> Mux40/3  "<v_0 x>"
  Constant21/1 -> Mux15/1
  Constant23/1 -> Mux13/2
  Bus Selector18/2 -> Mux38/2  "<t_0 y>"
  Mux13/1 -> Mux12/4
  Bus Selector25/3 -> Mux50/3  "<v_0 x>"
  Constant77/1 -> Traffic Object6/1
  Traffic Object9/1 -> Terminator9/1
  Bus Selector8/2 -> Mux14/2  "<t_0 y>"
  Traffic Object30/1 -> Terminator30/1
  Constant37/1 -> Mux23/2
  Mux23/1 -> Mux22/4
  Bus Selector6/3 -> Mux57/3  "<r_zyx z>"
  Traffic Object18/2 -> Bus Selector17/1
  Traffic Object8/2 -> Bus Selector6/1
  Bus Selector15/3 -> Mux28/3  "<r_zyx z>"
  Mux4/1 -> Mux1/4
  Constant16/1 -> Mux11/1
  Constant22/1 -> Mux4/1
  Traffic Object15/2 -> Bus Selector15/1
  Traffic Object9/2 -> Bus Selector7/1
  Traffic Object30/2 -> Bus Selector10/1
  Constant54/1 -> Traffic Object18/1
  Bus Selector9/1 -> Mux12/1  "<t_0 x>"
  Constant15/1 -> Traffic Object9/1
  Bus Selector26/2 -> Mux54/2  "<t_0 y>"
  Mux65/1 -> Mux64/9
  Bus Selector28/1 -> Mux16/1  "<t_0 x>"
  Constant32/1 -> Mux21/1
  Bus Selector10/2 -> Mux22/2  "<t_0 y>"
  Constant31/1 -> Traffic Object11/1
  Bus Selector9/2 -> Mux12/2  "<t_0 y>"
  Bus Selector20/2 -> Mux40/2  "<t_0 y>"
  Constant36/1 -> Mux21/2
  Mux20/1 -> [Traffic_Info_12]
  Constant26/1 -> Mux17/1
  Bus Selector24/4 -> Mux48/4  "<v_0 y>"
  Traffic Object7/2 -> Bus Selector8/1
  Bus Selector14/3 -> Mux30/3  "<r_zyx z>"
  Mux48/1 -> [Traffic_Info_25]
  Constant40/1 -> Mux25/2
  Traffic Object31/2 -> Bus Selector28/1
  Bus Selector11/3 -> Mux20/3  "<r_zyx z>"
  Traffic Object3/1 -> Terminator3/1
  [Traffic_Info_00] -> Mux59/1
  Bus Selector23/6 -> Mux44/6  "<a_0 y>"
  Mux17/1 -> Mux16/4
  Traffic Object5/2 -> Bus Selector4/1
  Bus Selector27/1 -> Mux52/1  "<t_0 x>"
  Mux33/1 -> Mux32/4
  [Traffic_Info_13] -> Mux59/14
  Constant46/1 -> Mux29/1
  [Traffic_Info_03] -> Mux59/4
  Bus Selector29/1 -> Mux60/1  "<t_0 x>"
  Constant38/1 -> Traffic Object13/1
  Mux38/1 -> [Traffic_Info_17]
  Constant61/1 -> Mux39/1
  Traffic Object8/1 -> Terminator8/1
  Constant95/1 -> Traffic Object28/1
  Bus Selector16/1 -> Mux32/1  "<t_0 x>"
  Bus Selector8/1 -> Mux14/1  "<t_0 x>"
  Bus Selector4/3 -> Mux5/3  "<r_zyx z>"
  Mux39/1 -> Mux38/4
  Traffic Object10/2 -> Bus Selector30/1
  Traffic Object29/1 -> Terminator29/1
  Constant52/1 -> Mux33/1
  Mux19/1 -> Mux18/4
  Bus Selector7/2 -> Mux10/2  "<t_0 y>"
  Bus Selector19/1 -> Mux36/1  "<t_0 x>"
  Bus Selector28/3 -> Mux16/3  "<r_zyx z>"
  Constant88/1 -> Mux56/1
  Constant34/1 -> Traffic Object30/1
  [Traffic_Info_09] -> Mux59/10
  Bus Selector16/2 -> Mux32/2  "<t_0 y>"
  Bus Selector18/1 -> Mux38/1  "<t_0 x>"
  Constant19/1 -> Mux13/1
  Bus Selector9/3 -> Mux12/3  "<r_zyx z>"
  Traffic Object14/1 -> Terminator14/1
  Constant63/1 -> Mux39/2
  Traffic Object29/2 -> Bus Selector9/1
  Traffic Object21/2 -> Bus Selector20/1
  Traffic Object16/2 -> Bus Selector18/1
  Bus Selector12/2 -> Mux24/2  "<t_0 y>"
  Traffic Object11/1 -> Terminator11/1
  Bus Selector6/1 -> Mux57/1  "<t_0 x>"
  Bus Selector12/1 -> Mux24/1  "<t_0 x>"
  Bus Selector27/6 -> Mux52/6  "<a_0 y>"
  Bus Selector21/2 -> Mux42/2  "<t_0 y>"
  Constant49/1 -> Mux29/2
  Mux27/1 -> Mux26/4
  Mux29/1 -> Mux28/4
  Traffic Object23/2 -> Bus Selector23/1
  Constant66/1 -> Mux8/2
  Mux30/1 -> [Traffic_Info_13]
  Constant42/1 -> Mux27/1
  Bus Selector27/3 -> Mux52/3  "<v_0 x>"
  Bus Selector13/1 -> Mux26/1  "<t_0 x>"
  [Traffic_Info_28] -> Mux59/29
  Mux42/1 -> [Traffic_Info_22]
  Bus Selector11/2 -> Mux20/2  "<t_0 y>"
  Mux5/1 -> [Traffic_Info_02]
  Traffic Object10/1 -> Terminator10/1
  Mux16/1 -> [Traffic_Info_10]
  Mux50/1 -> [Traffic_Info_26]
  Bus Selector21/1 -> Mux42/1  "<t_0 x>"
  Read CM Dict26/1 -> Mux48/8
  Mux34/1 -> [Traffic_Info_19]
  Constant20/1 -> Traffic Object7/1
  Bus Selector26/1 -> Mux54/1  "<t_0 x>"
  Bus Selector17/3 -> Mux34/3  "<r_zyx z>"
  Constant41/1 -> Traffic Object14/1
  Constant56/1 -> Mux35/1
  Bus Selector17/2 -> Mux34/2  "<t_0 y>"
  Traffic Object17/2 -> Bus Selector16/1
  Bus Selector10/1 -> Mux22/1  "<t_0 x>"
  Constant17/1 -> Mux11/2
  Mux21/1 -> Mux20/4
  Traffic Object27/2 -> Bus Selector27/1
  Mux31/1 -> Mux30/4
  Bus Selector31/5 -> Mux64/5  "<a_0 x>"
  [Traffic_Info_15] -> Mux59/16
  Traffic Object17/1 -> Terminator17/1
  Bus Selector12/3 -> Mux24/3  "<r_zyx z>"
  Mux46/1 -> [Traffic_Info_20]
  Bus Selector3/3 -> Mux1/3  "<r_zyx z>"
  [Traffic_Info_21] -> Mux59/22
  [Traffic_Info_02] -> Mux59/3
  Traffic Object19/2 -> Bus Selector19/1
  Bus Selector18/3 -> Mux38/3  "<r_zyx z>"
  Traffic Object16/1 -> Terminator16/1
  Traffic Object7/1 -> Terminator7/1
  Bus Selector30/3 -> Mux18/3  "<r_zyx z>"
  Constant51/1 -> Traffic Object17/1
  Bus Selector11/1 -> Mux20/1  "<t_0 x>"
  Bus Selector30/2 -> Mux18/2  "<t_0 y>"
  Bus Selector4/1 -> Mux5/1  "<t_0 x>"
  [Traffic_Info_07] -> Mux59/8
  [Traffic_Info_20] -> Mux59/21
  [Traffic_Info_27] -> Mux59/28
  Bus Selector13/3 -> Mux26/3  "<r_zyx z>"
  [Traffic_Info_17] -> Mux59/18
  Constant81/1 -> Traffic Object26/1
  Traffic Object20/1 -> Terminator20/1
  Mux44/1 -> [Traffic_Info_23]
  Bus Selector31/6 -> Mux64/6  "<a_0 y>"
  Constant91/1 -> Traffic Object3/1
  Mux47/1 -> Mux46/4
  Mux66/1 -> [Parking_Map_Boundary]
  Constant101/1 -> Mux68/2
  Mux69/1 -> Mux66/4
  Constant104/1 -> Mux67/1
  Constant99/1 -> Mux67/2
  Mux68/1 -> Mux66/3
  Constant100/1 -> Mux68/1
  Mux63/1 -> Mux66/1
  Constant102/1 -> Mux69/1
  Constant98/1 -> Mux63/1
  Constant103/1 -> Mux69/2
  Subsystem1/1(Traffic_Info) -> Goto75/1
  Mux67/1 -> Mux66/2
  Constant105/1 -> Mux63/2
  Matrix Concatenate/1 -> MATLAB Function9/2(traffic_info), MATLAB Function11/5(traffic_info)
  [Traffic_Info_28] -> Transpose7/1
  [Traffic_Info_27] -> Transpose6/1
  [Traffic_Info_26] -> Transpose5/1
  [Traffic_Info_25] -> Transpose4/1
  [Traffic_Info_24] -> Transpose3/1
  [Traffic_Info_23] -> Transpose2/1
  [Traffic_Info_22] -> Transpose1/1
  [Traffic_Info_21] -> Transpose/1
  [Ego_Gloabl_Y] -> Mux6/2
  [Ego_Global_X] -> Mux6/1
  [ego_lane_idx] -> MATLAB Function11/4(ego_lane_idx)
  [traffic_lane_idx] -> MATLAB Function11/6(traffic_lane_idx)
  [Ego_Yaw] -> MATLAB Function11/2(ego_yaw)
  [Ego_Velocity] -> MATLAB Function11/3(ego_vx)
  MATLAB Function11/1(target_speed) -> Rate Limiter/1
  MATLAB Function11/2(debug_dist) -> Scope8/1
  Mux6/1 -> Scope1/1, MATLAB Function11/1(ego_pos)
  From31/1 -> Vector Concatenate4/2
  From29/1 -> Vector Concatenate3/2
  [Ego_Gloabl_Y] -> Mux2/2
  [Global_Waypoints1] -> MATLAB Function9/3(wp1)
  From28/1 -> Vector Concatenate3/1
  [Global_Waypoints3] -> MATLAB Function9/5(wp3)
  MATLAB Function9/2(traffic_lane_idx) -> [traffic_lane_idx], Scope6/1
  [Ego_Global_X] -> Mux2/1
  From30/1 -> Vector Concatenate4/1
  [Global_Waypoints2] -> MATLAB Function9/4(wp2)
  Vector Concatenate4/1 -> Matrix Concatenate1/2
  From33/1 -> Vector Concatenate5/2
  MATLAB Function9/1(ego_lane_idx) -> [ego_lane_idx], Scope/1
  From32/1 -> Vector Concatenate5/1
  Vector Concatenate3/1 -> Matrix Concatenate1/1
  Vector Concatenate5/1 -> Matrix Concatenate1/3
  Mux2/1 -> MATLAB Function9/1(ego_pos)
  Read CM Dict8/1 -> [Ego_Yaw]
  Constant9/1 -> [Global_Waypoints3]
  Read CM Dict7/1 -> [Ego_Velocity]
  Read CM Dict5/1 -> [Ego_Global_X]
  Constant8/1 -> [Global_Waypoints2]
  Read CM Dict6/1 -> [Ego_Gloabl_Y]
  Constant6/1 -> [Global_Waypoints1]
  "MATLAB Function4 "/1(local_waypoints_) -> [Local_Points]
  Saturation1/1 -> Write CM Dict3/1, Write CM Dict4/1
  MATLAB Function3/1(lateral_error) -> [LateralError]
  Mux/1 -> "MATLAB Function4 "/2(vehicle_position)
  [Ego_Velocity] -> MATLAB Function3/2(velocity)
  [Ego_Global_X] -> Mux/1
  [Local_Points] -> MATLAB Function4/1(local_waypoints)
  Constant7/1 -> MATLAB Function3/3(lookahead_time)
  MATLAB Function4/1(poly_coeff) -> [Coefficients], Scope2/1
  [Global_Waypoints4] -> "MATLAB Function4 "/1(waypoints)
  [Coefficients] -> MATLAB Function3/1(poly_coeff)
  [Ego_Yaw] -> "MATLAB Function4 "/3(head)
  [Ego_Gloabl_Y] -> Mux/2
  Constant4/1 -> Goto29/1
  Read CM Dict4/1 -> Goto27/1
  Subsystem/1(Traffic_Info) -> Goto30/1
  Mux3/1 -> Reshape1/1
  Reshape1/1 -> Goto28/1
  Constant5/1 -> Mux3/2
  Constant10/1 -> Mux3/1
  Bus Selector2/4 -> Goto24/1  "<v_0 y>"
  Read CM Dict3/1 -> Goto20/1
  Bus Selector2/5 -> Goto25/1  "<a_0 x>"
  Bus Selector2/7 -> Goto19/1  "<r_zyx z>"
  Traffic Object2/1 -> Terminator2/1
  Constant3/1 -> Traffic Object2/1
  Bus Selector2/6 -> Goto26/1  "<a_0 y>"
  Bus Selector2/1 -> Goto21/1  "<t_0 x>"
  Traffic Object2/2 -> Bus Selector2/1
  Bus Selector2/2 -> Goto22/1  "<t_0 y>"
  Bus Selector2/3 -> Goto23/1  "<v_0 x>"
  Bus Selector1/2 -> Goto14/1  "<t_0 y>"
  Bus Selector1/3 -> Goto15/1  "<v_0 x>"
  Traffic Object1/2 -> Bus Selector1/1
  Constant2/1 -> Traffic Object1/1
  Bus Selector1/4 -> Goto16/1  "<v_0 y>"
  Traffic Object1/1 -> Terminator1/1
  Bus Selector1/7 -> Goto11/1  "<r_zyx z>"
  Bus Selector1/6 -> Goto18/1  "<a_0 y>"
  Bus Selector1/5 -> Goto17/1  "<a_0 x>"
  Bus Selector1/1 -> Goto13/1  "<t_0 x>"
  Read CM Dict2/1 -> Goto12/1
  Bus Selector/7 -> Goto10/1  "<r_zyx z>"
  Bus Selector/6 -> Goto9/1  "<a_0 y>"
  Bus Selector/5 -> Goto8/1  "<a_0 x>"
  Read CM Dict1/1 -> Goto2/1
  Bus Selector/2 -> Goto5/1  "<t_0 y>"
  Bus Selector/1 -> Goto3/1  "<t_0 x>"
  Traffic Object/2 -> Bus Selector/1
  Bus Selector/3 -> Goto6/1  "<v_0 x>"
  Traffic Object/1 -> Terminator/1
  Bus Selector/4 -> Goto7/1  "<v_0 y>"
  Constant/1 -> Goto4/1
  Read CM Dict/1 -> Goto1/1
  Constant1/1 -> Traffic Object/1
  Gain1/1 -> Sum1/1
  [Ego_Gloabl_Y] -> MATLAB Function/2(u2)
  [Ego_Global_X] -> MATLAB Function/1(u1)
  Switch/1 -> Add/1
  Add/1 -> PID Controller1/1
  [Ego_Velocity] -> Add/2
  Constant112/1 -> Gain2/1
  Gain2/1 -> Switch/1
  PID Controller1/1 -> Write CM Dict5/1
  [Target_speed2] -> Switch/3
  MATLAB Function/1(y) -> Scope3/1, Switch/2
  Rate Limiter/1 -> Scope4/1, [Target_speed2]

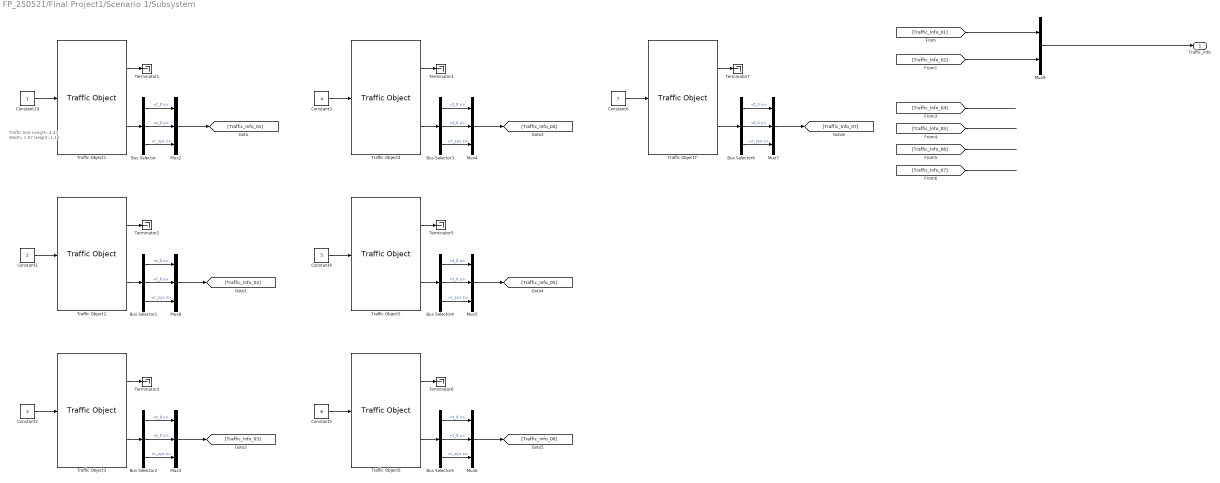
== system FP_250521/Final Project1/Scenario 1/Subsystem ==
  note: Traffic Size
      | Length: 4.47
      | Width: 1.97
      | Height: 1.12
  Bus Selector{,1..6} (7 alike) : BusSelector  OutputSignals=t_0 x,t_0 y,r_zyx z
  Constant1 : Constant  Value=2
  Constant10 : Constant
  Constant2 : Constant  Value=3
  Constant3 : Constant  Value=4
  Constant4 : Constant  Value=5
  Constant5 : Constant  Value=6
  Constant6 : Constant  Value=7
  Mux{2..8} (7 alike) : Mux  Inputs=3
  Mux9 : Mux  Inputs=2
  Terminator{1..7} (7 alike) : Terminator
  Traffic Object1 : CarMaker4SL/Traffic Object  xname=T01  ximode=Traffic Id  xstime=Inherited
      settings: SourceProductName=CarMaker4SL
  Traffic Object2 : CarMaker4SL/Traffic Object  xname=T02  ximode=Traffic Id  xstime=Inherited
      settings: SourceProductName=CarMaker4SL
  Traffic Object3 : CarMaker4SL/Traffic Object  xname=T03  ximode=Traffic Id  xstime=Inherited
      settings: SourceProductName=CarMaker4SL
  Traffic Object4 : CarMaker4SL/Traffic Object  xname=T04  ximode=Traffic Id  xstime=Inherited
      settings: SourceProductName=CarMaker4SL
  Traffic Object5 : CarMaker4SL/Traffic Object  xname=T05  ximode=Traffic Id  xstime=Inherited
      settings: SourceProductName=CarMaker4SL
  Traffic Object6 : CarMaker4SL/Traffic Object  xname=T06  ximode=Traffic Id  xstime=Inherited
      settings: SourceProductName=CarMaker4SL
  Traffic Object7 : CarMaker4SL/Traffic Object  xname=T07  ximode=Traffic Id  xstime=Inherited
      settings: SourceProductName=CarMaker4SL
  Traffic_Info : Outport
  wires:
  Constant10/1 -> Traffic Object1/1
  Traffic Object1/1 -> Terminator1/1
  Traffic Object2/1 -> Terminator2/1
  Constant1/1 -> Traffic Object2/1
  Constant2/1 -> Traffic Object3/1
  Traffic Object3/1 -> Terminator3/1
  Traffic Object4/1 -> Terminator4/1
  Constant3/1 -> Traffic Object4/1
  Constant4/1 -> Traffic Object5/1
  Traffic Object5/1 -> Terminator5/1
  Traffic Object6/1 -> Terminator6/1
  Constant5/1 -> Traffic Object6/1
  Constant6/1 -> Traffic Object7/1
  Traffic Object7/1 -> Terminator7/1
  [Traffic_Info_04] -> ?
  [Traffic_Info_05] -> ?
  [Traffic_Info_06] -> ?
  [Traffic_Info_07] -> ?
  Traffic Object1/2 -> Bus Selector/1
  Bus Selector/1 -> Mux2/1  "<t_0 x>"
  Bus Selector/2 -> Mux2/2  "<t_0 y>"
  Bus Selector/3 -> Mux2/3  "<r_zyx z>"
  Bus Selector1/2 -> Mux8/2  "<t_0 y>"
  Mux8/1 -> [Traffic_Info_02]
  Bus Selector1/1 -> Mux8/1  "<t_0 x>"
  Bus Selector1/3 -> Mux8/3  "<r_zyx z>"
  Traffic Object2/2 -> Bus Selector1/1
  Bus Selector2/2 -> Mux3/2  "<t_0 y>"
  Mux3/1 -> [Traffic_Info_03]
  Bus Selector2/1 -> Mux3/1  "<t_0 x>"
  Bus Selector2/3 -> Mux3/3  "<r_zyx z>"
  Traffic Object3/2 -> Bus Selector2/1
  Bus Selector3/2 -> Mux4/2  "<t_0 y>"
  Mux4/1 -> [Traffic_Info_04]
  Bus Selector3/1 -> Mux4/1  "<t_0 x>"
  Bus Selector3/3 -> Mux4/3  "<r_zyx z>"
  Traffic Object4/2 -> Bus Selector3/1
  Bus Selector4/2 -> Mux5/2  "<t_0 y>"
  Mux5/1 -> [Traffic_Info_05]
  Bus Selector4/1 -> Mux5/1  "<t_0 x>"
  Bus Selector4/3 -> Mux5/3  "<r_zyx z>"
  Traffic Object5/2 -> Bus Selector4/1
  Bus Selector5/2 -> Mux6/2  "<t_0 y>"
  Mux6/1 -> [Traffic_Info_06]
  Bus Selector5/1 -> Mux6/1  "<t_0 x>"
  Bus Selector5/3 -> Mux6/3  "<r_zyx z>"
  Traffic Object6/2 -> Bus Selector5/1
  Bus Selector6/2 -> Mux7/2  "<t_0 y>"
  Mux7/1 -> [Traffic_Info_07]
  Bus Selector6/1 -> Mux7/1  "<t_0 x>"
  Bus Selector6/3 -> Mux7/3  "<r_zyx z>"
  Traffic Object7/2 -> Bus Selector6/1
  Mux2/1 -> [Traffic_Info_01]
  [Traffic_Info_01] -> Mux9/1
  [Traffic_Info_02] -> Mux9/2
  Mux9/1 -> Traffic_Info/1
